simulink model "APF_CTL_VIS_Obs_2023a"  (R2023a)
settings: Solver=ode4  StartTime=0.0  StopTime=tsim  FixedStep=baseRate  RelTol=1e-6  AbsTol=1e-6
values from neighbouring files (symbols this model uses):
  A = [0 0 0 1 0 0 ... (first row only)    [CTL_NEW.m]    (also in UKF_SPOT.m = [1 0 0 dt 0 0)
  a = 25.028    [CTL_NEW.m]
  a1 = shape(1)    [Cardioid.m]    (also in Run_Initializer.m = 0.3)
  a2 = shape(2)    [Cardioid.m]    (also in Run_Initializer.m = 0.3)
  a3 = shape(3)    [Cardioid.m]    (also in Run_Initializer.m = 0.4)
  adadelta_epsilon = 1e-5    (= 1e-05)    [Run_Initializer.m]
  adadelta_gamma = 0.37    [Run_Initializer.m]
  adagrad_epsilon = 1e-8    (= 1e-08)    [Run_Initializer.m]
  adagrad_eta = 0.18    [Run_Initializer.m]
  adam_beta_1 = 0.99    [Run_Initializer.m]
  adam_beta_2 = 0.999    [Run_Initializer.m]
  adam_epsilon = 1e-2    (= 0.01)    [Run_Initializer.m]
  adam_eta = 0.0163    [Run_Initializer.m]
  adamax_beta_1 = 0.5    [Run_Initializer.m]
  adamax_beta_2 = 0.999    [Run_Initializer.m]
  adamax_eta = 0.014    [Run_Initializer.m]
  alpha_Black = 0.9    [UKF_SPOT.m]
  alpha_Blue = 0.9    [UKF_SPOT.m]
  Att_Mode = 0    [Run_Initializer.m]
  b1 = shape(4)    [Cardioid.m]    (also in Run_Initializer.m = 0.175)
  b2 = shape(5)    [Cardioid.m]    (also in Run_Initializer.m = 0.175)
  beta_Black = 2    [UKF_SPOT.m]
  beta_Blue = 20    [UKF_SPOT.m]
  Binv = inv(B)    [Run_Initializer.m]
  BLACK_end = [2, 1.4, deg2rad(368)]    [Run_Initializer.m]
  BLACK_ini = [2, 1.4, deg2rad(188), 0, 0, deg2rad(1.5)]    [Run_Initializer.m]
  BLUE_end = [1.3, 1.25, deg2rad(90)]    [Run_Initializer.m]
  BLUE_ini = [1.3, 1.25, deg2rad(270), 0, 0, deg2rad(-1.5)]    [Run_Initializer.m]
  drop_states_BLACK = BLACK_ini(1:3)    [Run_Initializer.m]
  drop_states_BLUE = BLUE_ini(1:3)    [Run_Initializer.m]
  drop_states_RED = RED_ini(1:3)    [Run_Initializer.m]
  dt = 0.01    [UKF_SPOT.m]
  end_time_black = 300    [Run_Initializer.m]
  end_time_blue = 300    [Run_Initializer.m]
  F_max = 0.22    [CTL_NEW.m]
  Gamma1_el = 0.12    [Run_Initializer.m]
  Gamma1_sh = 0.005    [Run_Initializer.m]
  Gamma1_wr = 0.025    [Run_Initializer.m]
  Gamma2_el = 5    [Run_Initializer.m]
  Gamma2_sh = 5    [Run_Initializer.m]
  Gamma2_wr = 5    [Run_Initializer.m]
  Gamma3_el = 10    [Run_Initializer.m]
  Gamma3_sh = 40    [Run_Initializer.m]
  Gamma3_wr = 40    [Run_Initializer.m]
  Gamma4_el = 0.039    [Run_Initializer.m]
  Gamma4_sh = 0.015    [Run_Initializer.m]
  Gamma4_wr = 0.029    [Run_Initializer.m]
  Gamma5_el = 800    [Run_Initializer.m]
  Gamma5_sh = 800    [Run_Initializer.m]
  Gamma5_wr = 800    [Run_Initializer.m]
  Gamma6_el = 0.000001    (= 1e-06)    [Run_Initializer.m]
  Gamma6_sh = 0.005    [Run_Initializer.m]
  Gamma6_wr = 0.02    [Run_Initializer.m]
  H = [1 0 0 0 0 0 ... (first row only)    [UKF_SPOT.m]
  home_states_BLACK = BLACK_ini(1:3)    [Run_Initializer.m]
  home_states_BLUE = BLUE_ini(1:3)    [Run_Initializer.m]
  home_states_RED = RED_ini(1:3)    [Run_Initializer.m]
  Hz = 0.01    [CTL_NEW.m]
  init_states_BLACK = BLACK_ini(1:3)    [Run_Initializer.m]
  init_states_BLUE = BLUE_ini(1:3)    [Run_Initializer.m]
  init_states_RED = RED_ini(1:3)    [Run_Initializer.m]
  J = IRED    [CTL_NEW.m]    (also in UKF_SPOT.m = 0.20184)
  k = lqr(A,B1,Q,R)    [CTL_NEW.m]
  k_1_0 = k(1,1)    [CTL_NEW.m]
  k_1_t_0 = k(3,3)    [CTL_NEW.m]
  k_2_0 = k(1,4)    [CTL_NEW.m]
  k_2_t_0 = k(3,6)    [CTL_NEW.m]
  K_a = diag([2 2 3.5])    [Run_Initializer.m]
  ka = 1    [Run_Initializer.m]
  Kd_elarm = 0.8    [Run_Initializer.m]
  Kd_sharm = 1.0    (= 1)    [Run_Initializer.m]
  Kd_t = 9.5    [CTL_NEW.m]    (also in Run_Initializer.m)
  Kd_wrarm = 0.6    [Run_Initializer.m]
  Kd_x = 28    [CTL_NEW.m]    (also in Run_Initializer.m)
  Kd_y = Kd_x    (= 28)    [CTL_NEW.m]    (also in Run_Initializer.m)
  Kp_elarm = 1.2    [Run_Initializer.m]
  Kp_sharm = 1.5    [Run_Initializer.m]
  Kp_t = 1    [CTL_NEW.m]    (also in Run_Initializer.m)
  Kp_wrarm = 2    [Run_Initializer.m]
  Kp_x = 3.5    [CTL_NEW.m]    (also in Run_Initializer.m)
  Kp_y = Kp_x    (= 3.5)    [CTL_NEW.m]    (also in Run_Initializer.m)
  kr = 2    [Run_Initializer.m]
  lambda1 = 0.4    [CTL_NEW.m]
  lambda12 = 0.4    [CTL_NEW.m]
  lambda12_t = 0.05    [CTL_NEW.m]
  lambda1_t = 0.05    [CTL_NEW.m]
  lambda2 = 0.4    [CTL_NEW.m]
  lambda2_t = 0.05    [CTL_NEW.m]
  lamda_Black = (alpha_Black^2)*(N + kappa_Black) - N    (= 15.06)    [UKF_SPOT.m]
  lamda_Blue = (alpha_Blue^2)*(N + kappa_Blue) - N    (= 6.96)    [UKF_SPOT.m]
  m = mRED    [CTL_NEW.m]    (also in UKF_SPOT.m = 11.21)
  method = 1    [UKF_SPOT.m]
  Method = 8    [Run_Initializer.m]
  momentum_eta = 0.7    [Run_Initializer.m]
  momentum_gamma = 0.7    [Run_Initializer.m]
  nesterov_eta = 0.6    [Run_Initializer.m]
  nesterov_gamma = 0.3    [Run_Initializer.m]
  Nmat = diag([1 1 1])    [Run_Initializer.m]
  p = 0.4    [CTL_NEW.m]
  P_b = diag([45 45 0])    [Run_Initializer.m]
  P_IC_Black = 0.2*eye(6)    [UKF_SPOT.m]
  P_IC_Blue = 0.2*eye(6)    [UKF_SPOT.m]
  p_t = 0.05    [CTL_NEW.m]
  psi = 1    [Run_Initializer.m]
  PWMFreq = 5    [Run_Initializer.m]
  Q = [w 0 0 0 0 0 ... (first row only)    [CTL_NEW.m]
  Q_a = diag([5, 5, 0])    [Run_Initializer.m]
  Q_b = diag([0.0125, 0.0125, 0.05])    [Run_Initializer.m]
  Q_Black = [0.0000005 0 0 0 0 0 ... (first row only)    [UKF_SPOT.m]
  Q_Blue = [0.000075 0 0 0 0 0 ... (first row only)    [UKF_SPOT.m]
  R = [r 0 0 ... (first row only)    [CTL_NEW.m]
  R_Black = [variance 0 0 ... (first row only)    [UKF_SPOT.m]
  R_Blue = [variance 0 0 ... (first row only)    [UKF_SPOT.m]
  r_hold = 0.427    [Run_Initializer.m]
  r_off = 0.165    [Run_Initializer.m]
  RED_ini = [2.7, 0.4, deg2rad(135+360), 0, 0, 0]    [Run_Initializer.m]
  Red_Rate = 0.025    [CTL_NEW.m]
  RMSprop_epsilon = 1e-8    (= 1e-08)    [Run_Initializer.m]
  RMSprop_eta = 0.025    [Run_Initializer.m]
  RMSprop_gamma = 0.9    [Run_Initializer.m]
  ... (+11 more)
undefined symbols (not defined in the file or in its folder): alpha, alpha_m, alphap, alphat, Am, b, b0, b3, baseRate, beta, Bm, c, Cm, d, DiscIntNeverNeededParam, Dm, drop_states_ARM, epsilon, F_Black_X_nominal, F_Black_Y_nominal, F_Blue_X_nominal, F_Blue_Y_nominal, F_red_X_nominal, F_red_Y_nominal, F_thrusters_BLACK, F_thrusters_BLUE, F_thrusters_RED, IBLACK, IBLUE, IDIST, IEE, IPROX, IRED, K, k1, k1t, k2, k2t, K_t, Kd_tb, Kd_tblue, Kd_tr, Kd_xb, Kd_xblue, Kd_xr, Kd_yb, Kd_yblue, Kd_yr, Kp_tb, Kp_tblue, Kp_tr, Kp_xb, Kp_xblue, Kp_xr, Kp_yb, Kp_yblue, Kp_yr, lamda ... (+34)
libraries: nvidiaSharedBlocks x10, MainLibrary x4, dspsigops x4, simulink x2, etargetslib x1
(part 14 of 15)

== matlab function APF_CTL_VIS_Obs_2023a/Phase #3: Experiment/Change RED Behavior/Sub-Phase #4/CTL/If Action Subsystem/Sat/MATLAB Function4 ==
  data: q2 input; u input; saturation output; F_max parameter; b parameter; m parameter; e parameter
function saturation = fcn(q2,u,F_max, b, m, e)

if u >= e
    u = e;
elseif u <= -1*e
    u = -1*e;
else
    u = u;
end

u = b*q2*m + u;

if u >= F_max
    u = F_max;
elseif u <= -1*F_max
    u = -1*F_max;
else
    u = u;
end

saturation = u;

== matlab function APF_CTL_VIS_Obs_2023a/Phase #3: Experiment/Change RED Behavior/Sub-Phase #4/CTL/If Action Subsystem/Sat/MATLAB Function5 ==
  data: q2 input; u input; saturation output; e parameter; T_max parameter; d parameter; J parameter
function saturation = fcn(q2,u,e, T_max, d, J)

if u >= e
    u = e;
elseif u <= -1*e
    u = -1*e;
else
    u = u;
end

u = d*q2*J + u;

if u >= T_max
    u = T_max;
elseif u <= -1*T_max
    u = -1*T_max;
else
    u = u;
end

saturation = u;

== matlab function APF_CTL_VIS_Obs_2023a/Phase #3: Experiment/Change RED Behavior/Sub-Phase #4/BLUE/Ryan's Transform ==
  data: Measurments input; Blue_Measurments_table_ref output; Red_States input; delta parameter
function Blue_Measurments_table_ref = RelitivetoTable(Measurments,Red_States,delta)
if anynan(Measurments)
    Blue_Measurments_table_ref = [NaN;NaN;NaN];
else

 Measurments(1,1) = Measurments(1);
 Measurments(2,1) = Measurments(2);
 Measurments = [Measurments; Red_States(3)];

%% This code is very scuffed, so I added lots of notes, feel free to change this
%% Size check
if size(Red_States,1) == 6 || size(Red_States,2) == 6
    Red_States = Red_States(1:3);
elseif size(Red_States,1) == 3 || size(Red_States,2) == 3
    % Nothin
else
    disp('Error with demensions of Red_States')
    disp('Please use 3 or 6 states')
    disp(':(')
end

if size(Measurments,1) == 3 || size(Measurments,2) == 3
    % Nothin
else
    disp('Error with demensions of Measurments')
    disp('VIS only gives 3 states, please only use 3 states')
    disp(':(')
end
Red_States(3) = mod(Red_States(3) + pi, 2*pi) - pi;

%% Rotation matrix scuffed (accounts for the location change of the docking cone) + Camera Offset of 3 deg
     c3 = [sin(Red_States(3) + delta*pi/180),  cos(Red_States(3) + delta*pi/180), 0;
          cos(Red_States(3) + delta*pi/180), -sin(Red_States(3) + delta*pi/180), 0;
          0,                     0,                    1];

%% Measurments in table ref frame
    Blue_Measurments_table_ref = c3*Measurments;

%% Vector addition
    Blue_Measurments_table_ref(1) = Blue_Measurments_table_ref(1) + Red_States(1); 
    Blue_Measurments_table_ref(2) =  -1*Blue_Measurments_table_ref(2) + Red_States(2); % Negative Y value accounting for "Left Hand Rule"

%% Angle addition
    Blue_Measurments_table_ref(3) = Red_States(3); % Setting this just to give an estimate

%% Wrapping Angle from -pi to pi
% Dont ask me why, its consistant with the SPOT inport from phasespace
% Dont belive me, look at this, angular velocity is being unwrapped, therefor, angle must be wrapped
% APF_Path_Planning_2023a/PhaseSpace Camera Code/Use Hardware to Obtain States
    % Black_Measurments_table_ref(3) = mod(Black_Measurments_table_ref(3) + pi, 2*pi) - pi;
end
end

== matlab function APF_CTL_VIS_Obs_2023a/Phase #3: Experiment/Change RED Behavior/Sub-Phase #4/CTL/Subsystem1/SAT_Angle1/MATLAB Function2 ==
  data: q2 input; q1 input; saturation output; c parameter; d parameter; J parameter
function saturation = fcn(q2,q1,c, d, J)

u = c*J*q1 + c*J*q2/d;

saturation = u;

== matlab function APF_CTL_VIS_Obs_2023a/Phase #3: Experiment/Change RED Behavior/Sub-Phase #4/CTL/Subsystem1/SAT_Angle1/MATLAB Function5 ==
  data: q2 input; u input; saturation output; e parameter; T_max parameter; d parameter; J parameter
function saturation = fcn(q2,u,e, T_max, d, J)

if u >= e
    u = e;
elseif u <= -1*e
    u = -1*e;
else
    u = u;
end

u = d*q2*J + u;

if u >= T_max
    u = T_max;
elseif u <= -1*T_max
    u = -1*T_max;
else
    u = u;
end

saturation = u;

== matlab function APF_CTL_VIS_Obs_2023a/Phase #3: Experiment/Change RED Behavior/Sub-Phase #4/CTL/Subsystem1/Subsystem/SAC Ctl/SAC Fns ==
  data: um input; u output; xm input; ey input; Ke_l input; Kx_l input; Ku_l input; Ke output; Kx output; Ku output; Kedot_l output; Kxdot_l output; Kudot_l output
function [u, Ke, Kx, Ku, Kedot_l, Kxdot_l, Kudot_l] = sac(um, xm, ey, Ke_l, Kx_l, Ku_l)

%%% Gains
gamma_l = [451300 0 0; 0 0 0; 0 0 0] ;
gamma_p = 3.5*[122500 0 0; 0 534500 0; 0 0 258000] ;
sigma_sac = 0.93 ;

%%% Ke
Kpe = ey*ey'*gamma_p(1,1) ;
Kedot_l = ey*ey'*gamma_l(1,1) - sigma_sac*Ke_l ;
Ke = Kpe + Ke_l ;

%%% Kx
Kpx = ey*xm'*gamma_p(2,2) ;
Kxdot_l = ey*xm'*gamma_l(2,2) ;
Kx = Kpx + Kx_l ;

%%% Ku
Kpu = ey*um'*gamma_p(3,3) ;
Kudot_l = ey*um'*gamma_l(3,3) ;
Ku = Kpu + Ku_l ;

%%% input
u = Ke*ey + Kx*xm + Ku*um ;

== matlab function APF_CTL_VIS_Obs_2023a/Phase #3: Experiment/Change RED Behavior/Sub-Phase #4/CTL/If Action Subsystem/DAC Controller3/Fx Gain Derivatives ==
  data: e_xdot input; k2_dot output; e_x input; k1_dot output; lambda1 parameter; lambda2 parameter; lambda12 parameter; p parameter
function [k2_dot, k1_dot]= fcn(e_xdot, e_x, lambda1, lambda2, lambda12, p)

k1_dot = -lambda1*p*e_x^2-(lambda1+p*lambda12)*e_x*e_xdot-lambda12*e_xdot^2;
k2_dot = -lambda12*p*e_x^2-(lambda12+p*lambda2)*e_x*e_xdot-lambda2*e_xdot^2;

== matlab function APF_CTL_VIS_Obs_2023a/Phase #3: Experiment/Change RED Behavior/Sub-Phase #4/CTL/If Action Subsystem/DAC Controller3/Fy Gain Derivatives ==
  data: k2_dot output; e_ydot input; e_y input; k1_dot output; lambda1 parameter; lambda2 parameter; lambda12 parameter; p parameter
function [k2_dot, k1_dot]= fcn(e_ydot, e_y, lambda1, lambda2, lambda12, p)

k1_dot = -lambda1*p*e_y^2-(lambda1+p*lambda12)*e_y*e_ydot-lambda12*e_ydot^2;
k2_dot = -lambda12*p*e_y^2-(lambda12+p*lambda2)*e_y*e_ydot-lambda2*e_ydot^2;

== matlab function APF_CTL_VIS_Obs_2023a/Phase #3: Experiment/Change RED Behavior/Sub-Phase #4/CTL/Subsystem1/SAT_Angle1/Torque Gain Derivatives ==
  data: e_t input; e_tdot input; k1_dot output size=1; k2_dot output size=1; lambda1_t parameter; lambda2_t parameter; lambda12_t parameter; p_t parameter
function [k1_dot, k2_dot]= fcn(e_t, e_tdot, lambda1_t, lambda2_t, lambda12_t, p_t)
k1_dot = -lambda1_t*p_t*e_t^2-(lambda1_t+p_t*lambda12_t)*e_t*e_tdot-lambda12_t*e_tdot^2;
k2_dot = -lambda12_t*p_t*e_t^2-(lambda12_t+p_t*lambda2_t)*e_t*e_tdot-lambda2_t*e_tdot^2;

== matlab function APF_CTL_VIS_Obs_2023a/Phase #3: Experiment/Change RED Behavior/Sub-Phase #4/CTL/If Action Subsystem/DAC Controller3/Torque Gain Derivatives ==
  data: e_t input; e_tdot input; k1_dot output size=1; k2_dot output size=1; lambda1_t parameter; lambda2_t parameter; lambda12_t parameter; p_t parameter
function [k1_dot, k2_dot]= fcn(e_t, e_tdot, lambda1_t, lambda2_t, lambda12_t, p_t)
k1_dot = -lambda1_t*p_t*e_t^2-(lambda1_t+p_t*lambda12_t)*e_t*e_tdot-lambda12_t*e_tdot^2;
k2_dot = -lambda12_t*p_t*e_t^2-(lambda12_t+p_t*lambda2_t)*e_t*e_tdot-lambda2_t*e_tdot^2;

== matlab function APF_CTL_VIS_Obs_2023a/Phase #3: Experiment/Change RED Behavior/Sub-Phase #4/BLUE/Subsystem/MATLAB Function ==
  data: u1 input; y output; u2 input
function y = fcn(u1,u2)
if abs(u1(1) - u2(1)) < 1e-10
    y = [NaN;NaN];
else
    y = u1;
end
if u1 < 1e-10
    y = [NaN;NaN];
end

== matlab function APF_CTL_VIS_Obs_2023a/Phase #3: Experiment/Change RED Behavior/Sub-Phase #4/BLUE/UKF_New/MATLAB Function2 ==
  data: no_IC output; States output; P_K output; Reject_Sum output; Reject output; Measurments input; Force input; States_k1 input; P_K1 input; lamda_Blue parameter; J parameter; m parameter; dt parameter; Q_Blue parameter; alpha_Blue parameter; beta_Blue parameter; H parameter; R_Blue parameter; thresh_Blue parameter; method parameter; Reject_sumk1 input; Reject_k1 input; thresh_Factor_Blue parameter
function [no_IC,States,P_K,Reject_Sum,Reject] = UKF(Measurments,Force,States_k1,P_K1, lamda_Blue, J, m, dt, Q_Blue, alpha_Blue, beta_Blue, H, R_Blue,thresh_Blue, method,Reject_sumk1,Reject_k1, thresh_Factor_Blue)
%% Block diagram got messy so i put it all in one block
if isempty(Force)
    Force = [0;0;0];
end

%% Inital position
if all(States_k1 == 0) || anynan(States_k1)
    if anynan(Measurments)
        States = NaN(6,1);
        no_IC = 1;
        P_K = P_K1;
        Reject_Sum = 0;
        Reject = 0;
    else
        States = [Measurments;zeros(3,1)];
        no_IC = 0;
        P_K = P_K1;
        Reject_Sum = 0;
        Reject = 0;
    end
else
    no_IC = 0;

    X_Cal = fcn1(States_k1,P_K1,lamda_Blue,method);
    
    X_Cal_k1 = fcn2(Force,X_Cal,J,m,dt);
    
    [w_m,w_c,X_tilda_k,P_K1] = fcn3(X_Cal_k1,lamda_Blue, Q_Blue, alpha_Blue, beta_Blue);
    
    [Z_Bar,Z_Cal] = fcn4(X_Cal_k1, w_m,H);
    
    [P_xz_k,P_z_k] = fcn5(Z_Bar,Z_Cal,w_c,X_tilda_k,X_Cal,R_Blue);
    
    K_k = fcn6(P_xz_k,P_z_k);
    
    Z_k = fcn7(Measurments);

    [thresh_Dynamic,Reject_Sum] = Dyn_Thresh(thresh_Blue,Reject_k1,thresh_Factor_Blue,Reject_sumk1);
    
    Reject = fcn8(Z_k,Z_Bar,P_z_k,thresh_Dynamic);
    
    States = fcn9(Z_k,Reject,X_tilda_k,Z_Bar,K_k);
    
    P_K = fcn10(P_K1,P_z_k,K_k,Reject);
end
end

function X_Cal = fcn1(x_tilda_k,P_k,lamda,method)
%% Calculate size of sigma var
sz = 6;
N = 2*sz + 1;
X_Cal = zeros(sz,N);

%% Calculate initial sigma point
X_Cal(:,1) = x_tilda_k;

%% Calculate sigma distance
sigma = (6 + lamda)*P_k;
sigma = Cholesky_Decomposition(sigma,method);

%% Calculate Sigma Points
% Positive points
for i = 2:1:((N-1)/2) + 1
    fill = zeros(size(x_tilda_k));
    fill(i-1,1) = sigma(i-1,i-1);
    X_Cal(:,i) = x_tilda_k + fill;
end
% Negative Points
j = 1;
for i = N + 1 - ((N-1)/2):1:N
    fill = zeros(size(x_tilda_k));
    fill(j,1) = sigma(j,j);
    X_Cal(:,i) = x_tilda_k - fill;
    j = j + 1;
end
end

function L = Cholesky_Decomposition(mat,method)

%% Getting size of matrix
[row,col] = size(mat);

%% Make sure matrix can be decomposed
if ~isequal(size(mat), size(mat'))
    error('Input matrix must be symmetric');
end

if any(eig(mat) <= 0)
    % error('Input matrix must be positive definite'); %% Added Error
    % Handling
    mat = NearPositiveDefinite(mat,method);
end

%% Pre allocating Space
L = zeros(row,col);

% Perform Cholesky decomposition
    for i = 1:col
        % Compute the diagonal element
        L(i, i) = sqrt(mat(i, i) - sum(L(i, 1:i-1).^2));
        
        % Compute the elements below the diagonal
        for j = i+1:col
            L(j, i) = (mat(j, i) - sum(L(j, 1:i-1).*L(i, 1:i-1))) / L(i, i);
        end
    end
end

function A_P = NearPositiveDefinite(A,method)
%% Method 1 (Symmetric Polar Factor)
%% Method 2 (Eigenvalue Recomposition)
    % enforce symmetry
    if isreal(A)
        B = 0.5*(A + A');
    else
        B = 0.5*(A + A');
        B = real(B) + 1i*hermSign(B).*imag(B);
    end

    if method == 1
        [~,~,U] = svd(B);
        H = U*U';
        A = (B + H)/2;

    elseif method == 2
        % Eigenvalue recomposition with modification for complex matrices
        [V,D] = eig(B);
        if isreal(A)
            D = max(real(D), 0); % Ensure real part of eigenvalues is non-negative
        else
            % For complex matrices, ensure positive semidefinite
            D = max(D, 0); % Ensure eigenvalues are non-negative
            V = real(V); % Take the real part of eigenvectors
        end
        A = real(V)*real(D)*real(V)'; % Now this really real product really should be really real right?
    else
        error('Please select proper method for Near Positive Definite Iteration')
    end

    % enforce symmetry again
    A_P = 0.5*(A + A');

    % Iteration
    i = 1;
    j = 0;
    max_iterations = 1000; % Maximum iterations allowed before increment starts increasing exponentially
    large_j_threshold = 500; % Threshold value for j to start increasing increment exponentially

    while i ~= 0
        [~,i] = chol(A_P);
        j = j + 1;
        if i ~= 0 % if close, add a multiple of the identity scaled by the smallest eigenvalue
            eig_min = min(eig(A_P));
            if j <= large_j_threshold
                increment = (-real(eig_min)*j.^2 + eps(real(eig_min)))*eye(size(A));
            else
                % Increase increment exponentially
                increment = (abs(real(eig_min))*j.^2 + eps(real(eig_min)))*exp(0.1*(j - large_j_threshold))*eye(size(A));
            end
            A_P = A_P + increment;
        end
        if j > max_iterations % If j exceeds the maximum allowed iterations, break the loop
            break;
        end
    end
end

function X_Cal_k1  = fcn2( F, X_Cal_k, J, m, dt)
%% Pre-Define
X_Cal_k1 = zeros(size(X_Cal_k));
%% System Dynamics
A = [eye(3), eye(3)*dt;
    zeros(3), eye(3)];

B = [eye(2)*(dt^2)/(2*m), zeros(2,1);
     0,0, (dt^2)/(2*J);
     eye(2)*(dt)/(m), zeros(2,1);
     0,0, (dt)/(J)];

%% State propigation
f = size(X_Cal_k,2);
for i = 1:1:f
    X_Cal_k1(:,i) = A*X_Cal_k(:,i) + B*F; 
end
end

function [w_m,w_c,X_tilda_k,P_K] = fcn3(X_Cal_k1,lamda, Q, alpha, beta)
%% Sigma weights
sz = size(X_Cal_k1,2);
N = 6;

%% For non modifyed variation
% w_0 = kappa/(N + kappa);
% w_i = 1/(2*(N + kappa));
% w = w_i*ones(1,N);
% w(1,1) = w_0;

%% Additional step - Sigma Points Weights
w_m_0 = lamda/(N + lamda);
w_c_0 = (lamda/(N + lamda)) + beta + (1 - alpha^2);
w_i = 1/(2*(N + lamda));

w = w_i*ones(1,sz-1);
w_m = [w_m_0, w];
w_c = [w_c_0, w];

w_m = diag(w_m);
w_c = diag(w_c);

%% State Prediction
X_tilda_k = X_Cal_k1*w_m;
X_tilda_k = sum(X_tilda_k,2);


%% Covariance Prediction
P_K = (X_Cal_k1 - X_tilda_k)*w_c*(X_Cal_k1 - X_tilda_k)' + Q;

end

function [Z_Bar,Z_Cal] = fcn4(x_Cal_k1, w_m,H)
%% calc Z_Cal
N = size(x_Cal_k1,2);
Z_Cal = zeros(3,N);
for i = 1:1:N
    Z_Cal(:,i) = H*x_Cal_k1(:,i);
end

%% Calc Z_Bar
Z_Bar = Z_Cal*w_m;
Z_Bar = sum(Z_Bar,2);
end

function [P_xz_k,P_z_k] = fcn5(Z_Bar,Z_Cal,w_c,x_tilda_k1,X_Cal,R)
%% calc P_z
P_z_k = (Z_Cal - Z_Bar)*w_c*(Z_Cal - Z_Bar)' + R;

%% calc P_xz
P_xz_k = (X_Cal - x_tilda_k1)*w_c*(Z_Cal - Z_Bar)';
end

function K_k = fcn6(P_xz_k,P_z_k)
K_k = (P_xz_k)*P_z_k';
end

function Z_k = fcn7(z_k)
    %% Assuming that all states are given or no states are given
    if anynan(z_k)
        Z_k = 1000*ones(3,1);
    else
    Z_k = z_k;
    end
end

function  Reject = fcn8(Z_k,Z_Bar,P_z_k,thresh)
%% Calc Mahalanobis Distance
D_square = (transpose(Z_k - Z_Bar))*P_z_k*(Z_k - Z_Bar);
% mahalanobis_d = sqrt(D_square);

%% Determine if data should be rejected
if D_square < thresh
    Reject = 0;
else
    Reject = 1;
end
end

function [x] = fcn9(z,Reject,X_tilda_k,z_bar,K_k)
%% State estimate
    if Reject == 0
        x = X_tilda_k + K_k*(z - z_bar);
    else
        x = X_tilda_k;
    end
end

function P_K = fcn10(P_k1,P_z_k,K_k,Reject)
if Reject == 0
    P_K = P_k1 - (K_k*P_z_k)*K_k';
else
    P_K = P_k1;
end
end


function [thresh_Dynamic,Reject_Sum] = Dyn_Thresh(thresh_Black,Reject_k1,thresh_Factor_Black,Reject_sumk1)
if Reject_k1 == 1    
    Reject_Sum = Reject_sumk1 + 1;
    thresh_Dynamic = thresh_Black + Reject_Sum*thresh_Factor_Black;
else 
    Reject_Sum = 0;
    thresh_Dynamic = thresh_Black;
end
end

== matlab function APF_CTL_VIS_Obs_2023a/Thruster Control Code/Change RED Behavior/Calculate Thruster ON//OFF/MATLAB Function11 ==
  data: H output; thruster_dist2CG_RED parameter; F_red_X_nominal parameter; thrust_decay_factor input; F_red_Y_nominal parameter
function H   = MakeHWithDecay(thruster_dist2CG_RED,F_red_X_nominal, thrust_decay_factor, F_red_Y_nominal)


adjusted_thruster_dist2CG_RED = [thruster_dist2CG_RED(1);
                                 thruster_dist2CG_RED(2);
                                 thruster_dist2CG_RED(3);
                                 thruster_dist2CG_RED(4);
                                 thruster_dist2CG_RED(5);
                                 thruster_dist2CG_RED(6);
                                 thruster_dist2CG_RED(7);
                                 thruster_dist2CG_RED(8)];
                                 


Vec1 = [ -1
         -1
          0 
          0
          1
          1
          0
          0 ];
      
Vec2 = [  0
          0
          1
          1
          0
          0
         -1
         -1 ];
     
Vec3 = adjusted_thruster_dist2CG_RED./1000;

Mat1 = [Vec1, Vec2, Vec3]';

F_thrusters_RED = [F_red_X_nominal*thrust_decay_factor; F_red_X_nominal*thrust_decay_factor; F_red_Y_nominal*thrust_decay_factor; F_red_Y_nominal*thrust_decay_factor; F_red_X_nominal*thrust_decay_factor; F_red_X_nominal*thrust_decay_factor; F_red_Y_nominal*thrust_decay_factor; F_red_Y_nominal*thrust_decay_factor];

Mat2 = diag((F_thrusters_RED./2));

H    = Mat1*Mat2;

end

== matlab function APF_CTL_VIS_Obs_2023a/Phase #3: Experiment/Change RED Behavior/Sub-Phase #4/BLACK/Subsystem/MATLAB Function ==
  data: u1 input; y output; u2 input
function y = fcn(u1,u2)
if abs(u1(1) - u2(1)) < 1e-10
    y = [NaN;NaN;NaN];
else
    y = u1;
end

== matlab function APF_CTL_VIS_Obs_2023a/Simulate Plant Dynamics/RED and ARM Dynamics/RED + ARM/RED + ARM Dynamics/Inertia Function 1 ==
  data: mRED parameter; IRED parameter; Phi parameter; b0 parameter; a1 parameter; b1 parameter; a2 parameter; b2 parameter; a3 parameter; b3 parameter; mPROX parameter; mDIST parameter; mEE parameter; IPROX parameter; IDIST parameter; InertiaS output; x input; IEE parameter
function InertiaS = InertiaFunc3LINK(mRED, IRED, Phi, b0, a1, b1, a2, b2, a3, b3, mPROX, mDIST, mEE, IPROX, IDIST, x, IEE)

    q0 = x(3);
    q1 = x(4);
    q2 = x(5);
    q3 = x(6);
    
    t2 = a1+b1;
    t3 = a1.*mPROX;
    t4 = mDIST.*t2;
    t5 = mEE.*t2;
    t6 = q0+q1;
    t7 = cos(t6);
    t8 = t3+t4+t5;
    t9 = a2.*mDIST;
    t10 = a2+b2;
    t11 = mEE.*t10;
    t12 = q0+q1+q2;
    t13 = cos(t12);
    t14 = t9+t11;
    t15 = q0+q1+q2+q3;
    t16 = cos(t15);
    t17 = mRED+mPROX+mDIST+mEE;
    t18 = b0.*mPROX;
    t19 = b0.*mDIST;
    t20 = b0.*mEE;
    t21 = t18+t19+t20;
    t22 = (pi/2-Phi)+q0;
    t23 = sin(t6);
    t24 = sin(t12);
    t25 = sin(t15);
    t26 = a2.*mEE;
    t27 = b2.*mEE;
    t28 = t9+t26+t27;
    t29 = sin(t22);
    t86 = t7.*t8;
    t87 = t13.*t14;
    t88 = a3.*mEE.*t16;
    t30 = -t86-t87-t88-t21.*t29;
    t31 = cos(t22);
    t32 = t21.*t31;
    t89 = t8.*t23;
    t90 = t14.*t24;
    t91 = a3.*mEE.*t25;
    t33 = t32-t89-t90-t91;
    t34 = a1.^2;
    t35 = a2.^2;
    t36 = b0.^2;
    t37 = b1.^2;
    t38 = a1.*a2.*mDIST.*2.0;
    t39 = a1.*a2.*mEE.*2.0;
    t40 = a2.*b1.*mDIST.*2.0;
    t41 = a1.*b2.*mEE.*2.0;
    t42 = a2.*b1.*mEE.*2.0;
    t43 = b1.*b2.*mEE.*2.0;
    t44 = t38+t39+t40+t41+t42+t43;
    t45 = cos(q2);
    t46 = t44.*t45;
    t47 = a2.*a3.*mEE.*2.0;
    t48 = a3.*b2.*mEE.*2.0;
    t49 = t47+t48;
    t50 = cos(q3);
    t51 = t49.*t50;
    t52 = a1.*a3.*mEE.*2.0;
    t53 = a3.*b1.*mEE.*2.0;
    t54 = t52+t53;
    t55 = q2+q3;
    t56 = cos(t55);
    t57 = t54.*t56;
    t58 = (pi/2-Phi)-q1;
    t59 = sin(t58);
    t60 = -(pi/2-Phi)+q1+q2;
    t61 = sin(t60);
    t62 = -(pi/2-Phi)+q1+q2+q3;
    t63 = sin(t62);
    t64 = mPROX.*t34;
    t65 = mDIST.*t34;
    t66 = mEE.*t34;
    t67 = mDIST.*t35;
    t68 = mEE.*t35;
    t69 = a3.^2;
    t70 = mEE.*t69;
    t71 = mDIST.*t37;
    t72 = mEE.*t37;
    t73 = b2.^2;
    t74 = mEE.*t73;
    t75 = a1.*b1.*mDIST.*2.0;
    t76 = a1.*b1.*mEE.*2.0;
    t77 = a2.*b2.*mEE.*2.0;
    t78 = a2.*b0.*mDIST;
    t79 = a2.*b0.*mEE;
    t80 = b0.*b2.*mEE;
    t81 = t78+t79+t80;
    t82 = a1.*a3.*mEE;
    t83 = a3.*b1.*mEE;
    t84 = t82+t83;
    t85 = t56.*t84;
    t92 = a1.*b0.*mPROX;
    t93 = a1.*b0.*mDIST;
    t94 = a1.*b0.*mEE;
    t95 = b0.*b1.*mDIST;
    t96 = b0.*b1.*mEE;
    t97 = t92+t93+t94+t95+t96;
    t98 = t59.*t97;
    t112 = t61.*t81;
    t113 = a3.*b0.*mEE.*t63;
    t99 = IPROX+IDIST+IEE+t46+t51+t57+t64+t65+t66+t67+t68+t70+t71+t72+t74+t75+t76+t77+t98-t112-t113;
    t100 = a1.*a2.*mDIST;
    t101 = a1.*a2.*mEE;
    t102 = a2.*b1.*mDIST;
    t103 = a1.*b2.*mEE;
    t104 = a2.*b1.*mEE;
    t105 = b1.*b2.*mEE;
    t106 = t100+t101+t102+t103+t104+t105;
    t107 = t45.*t106;
    t108 = a2.*a3.*mEE;
    t109 = a3.*b2.*mEE;
    t110 = t108+t109;
    t111 = t50.*t110;
    t114 = IDIST+IEE+t51+t67+t68+t70+t74+t77+t85+t107;
    t115 = IEE+t70+t85+t111;
    t116 = IEE+t70+t111;
    InertiaS = reshape([t17,0.0,t30,-t86-t87-t88,-t88-t13.*t28,-t88,0.0,t17,t33,-t89-t90-t91,-t91-t24.*t28,-t91,t30,t33,IRED+IPROX+IDIST+IEE+t46+t51+t57+t64+t65+t66+t67+t68+t70+t71+t72+t74+t75+t76+t77+t59.*(a1.*b0.*mPROX.*2.0+a1.*b0.*mDIST.*2.0+a1.*b0.*mEE.*2.0+b0.*b1.*mDIST.*2.0+b0.*b1.*mEE.*2.0)+mPROX.*t36+mDIST.*t36+mEE.*t36-t61.*(a2.*b0.*mDIST.*2.0+a2.*b0.*mEE.*2.0+b0.*b2.*mEE.*2.0)-a3.*b0.*mEE.*t63.*2.0,t99,IDIST+IEE+t51+t67+t68+t70+t74+t77+t85+t107-t112-t113,IEE+t70+t85+t111-t113,-t7.*t8-t13.*t14-a3.*mEE.*t16,-t8.*t23-t14.*t24-a3.*mEE.*t25,t99,IPROX+IDIST+IEE+t46+t51+t57+t64+t65+t66+t67+t68+t70+t71+t72+t74+t75+t76+t77,t114,t115,-t13.*t28-a3.*mEE.*t16,-t24.*t28-a3.*mEE.*t25,IDIST+IEE+t51+t67+t68+t70+t74+t77+t85+t107-t61.*t81-a3.*b0.*mEE.*t63,t114,IDIST+IEE+t51+t67+t68+t70+t74+t77,t116,-a3.*mEE.*t16,-a3.*mEE.*t25,IEE+t70+t85+t111-a3.*b0.*mEE.*t63,t115,t116,IEE+t70],[6,6]);
end

== matlab function APF_CTL_VIS_Obs_2023a/Thruster Control Code/Change RED Behavior/Calculate Thruster ON//OFF/MATLAB Function7 ==
  data: H output; thruster_dist2CG_RED parameter; F_red_X_nominal parameter; thrust_decay_factor input; F_red_Y_nominal parameter
function H   = MakeHWithDecay(thruster_dist2CG_RED,F_red_X_nominal, thrust_decay_factor, F_red_Y_nominal)


adjusted_thruster_dist2CG_RED = [thruster_dist2CG_RED(1);
                                 thruster_dist2CG_RED(2);
                                 thruster_dist2CG_RED(3);
                                 thruster_dist2CG_RED(4);
                                 thruster_dist2CG_RED(5);
                                 thruster_dist2CG_RED(6);
                                 thruster_dist2CG_RED(7);
                                 thruster_dist2CG_RED(8)];
                                 


Vec1 = [ -1
         -1
          0 
          0
          1
          1
          0
          0 ];
      
Vec2 = [  0
          0
          1
          1
          0
          0
         -1
         -1 ];
     
Vec3 = adjusted_thruster_dist2CG_RED./1000;

Mat1 = [Vec1, Vec2, Vec3]';

F_thrusters_RED = [F_red_X_nominal*thrust_decay_factor; F_red_X_nominal*thrust_decay_factor; F_red_Y_nominal*thrust_decay_factor; F_red_Y_nominal*thrust_decay_factor; F_red_X_nominal*thrust_decay_factor; F_red_X_nominal*thrust_decay_factor; F_red_Y_nominal*thrust_decay_factor; F_red_Y_nominal*thrust_decay_factor];

Mat2 = diag((F_thrusters_RED));

H    = Mat1*Mat2;

end

== matlab function APF_CTL_VIS_Obs_2023a/Simulate Plant Dynamics/BLACK Dynamics/BLACK Dynamics Model/MATLAB Function ==
  data: control_inputs input; x_ddot output; mBLACK parameter; IBLACK parameter
function x_ddot = BLACK_dynamics(control_inputs, mBLACK, IBLACK)

%#codegen
% Fully define the size of x_ddot() for code generation:
x_ddot     = zeros(3,1);

% Extract the control inputs from the control_input vector:
Fx        = control_inputs(1);              % [N]
Fy        = control_inputs(2);              % [N]
Tz        = control_inputs(3);              % [N.m]

% Calculate the state acceleration vector:
x_ddot(1) = Fx/mBLACK;                      % [m/s^2]
x_ddot(2) = Fy/mBLACK;                      % [m/s^2]
x_ddot(3) = Tz/IBLACK;                      % [rad/s^2]

end

== matlab function APF_CTL_VIS_Obs_2023a/Simulate Plant Dynamics/BLUE Dynamics/BLUE  Dynamics Model/MATLAB Function ==
  data: control_inputs input; x_ddot output; mBLUE parameter; IBLUE parameter
function x_ddot = BLUE_dynamics(control_inputs, mBLUE, IBLUE)%#codegen
% Fully define the size of x_ddot() for code generation:
x_ddot     = zeros(3,1);

% Extract the control inputs from the control_input vector:
Fx        = control_inputs(1);              % [N]
Fy        = control_inputs(2);              % [N]
Tz        = control_inputs(3);              % [N.m]

% Calculate the state acceleration vector:
x_ddot(1) = Fx/mBLUE;                      % [m/s^2]
x_ddot(2) = Fy/mBLUE;                      % [m/s^2]
x_ddot(3) = Tz/IBLUE;                      % [rad/s^2]

end

== matlab function APF_CTL_VIS_Obs_2023a/Simulate Plant Dynamics/BLUE Dynamics/Sample and Hold Data to Match PhaseSpace (BLUE)/MATLAB Function ==
  data: TIME input; y output; SERVER input
function y = fcn(TIME, SERVER)

if mod(TIME,SERVER) == 0
    y = 1;
else
    y = 0;
end

== matlab function APF_CTL_VIS_Obs_2023a/Simulate Plant Dynamics/RED and ARM Dynamics/RED Only/RED Dynamics/RED Dynamics Model/MATLAB Function ==
  data: control_inputs input; x_ddot output; mRED parameter; IRED parameter
    function x_ddot = RED_dynamics(control_inputs, mRED, IRED)
    
        %#codegen
        % Fully define the size of x_ddot() for code generation:
        x_ddot     = zeros(3,1);
        
        % Extract the servicer model parameters from the model_param vector defined
        % in initialize.m:
        
        % Extract the control inputs from the control_input vector:
        Fx        = control_inputs(1);              % [N]
        Fy        = control_inputs(2);              % [N]
        Tz        = control_inputs(3);              % [N.m]
        
        % Calculate the state acceleration vector:
        x_ddot(1) = Fx/mRED;                      % [m/s^2]
        x_ddot(2) = Fy/mRED;                      % [m/s^2]
        x_ddot(3) = Tz/IRED;                      % [rad/s^2]
    
    end

== matlab function APF_CTL_VIS_Obs_2023a/Phase #2: Initial Position/Change RED Behavior/MATLAB Function2 ==
  data: error input; error_d input; u output; K_lqr parameter
function u = fcn(error,error_d,K_lqr)




u = K_lqr*([error(1);error(2);error(3);error_d(1);error_d(2);error_d(3)]);

end

== matlab function APF_CTL_VIS_Obs_2023a/Phase #3: Experiment/Change RED Behavior/Sub-Phase #4/GDC/APF/GDC/MATLAB Function ==
  data: phi_tot output; phi_tot_grad output; state_red input; state_black input size=[6 1]; state_blue input; u output size=[3 1]; shape parameter; ka parameter; kr parameter; Q_a parameter; Q_b parameter; P_b parameter; r_hold parameter; Binv parameter; K_a parameter; psi parameter; sigma parameter; r_off parameter; Nmat parameter; state_desired output; IsBlue input
function [phi_tot,phi_tot_grad,u,state_desired] = fcn(state_red,state_black,state_blue,shape,ka,kr,Q_a,Q_b,P_b,r_hold,Binv,K_a,psi,sigma,r_off,Nmat,IsBlue)

[phi_tot,phi_tot_grad,u,state_desired] = APF_func_Maybe_Obstacle(state_red,state_black,state_blue,shape,ka,kr,Q_a,Q_b,P_b,r_hold,Binv,K_a,psi,sigma,r_off,Nmat,IsBlue);

== matlab function APF_CTL_VIS_Obs_2023a/Thruster Control Code/Change BLACK Behavior/Calculate Thruster ON//OFF/MATLAB Function ==
  data: H output; thruster_dist2CG_BLACK parameter; F_thrusters_BLACK parameter
function H = MakeH(thruster_dist2CG_BLACK,F_thrusters_BLACK)

Vec1 = [ -1
         -1
          0 
          0
          1
          1
          0
          0 ];
      
Vec2 = [  0
          0
          1
          1
          0
          0
         -1
         -1 ];
     
Vec3 = thruster_dist2CG_BLACK./1000;

Mat1 = [Vec1, Vec2, Vec3]';

Mat2 = diag((F_thrusters_BLACK./2));

H    = Mat1*Mat2;

end

== matlab function APF_CTL_VIS_Obs_2023a/Thruster Control Code/Change BLUE Behavior/Calculate Thruster ON//OFF/MATLAB Function1 ==
  data: H output; thruster_dist2CG_BLUE parameter; F_Blue_X_nominal parameter; thrust_decay_factor input; F_Blue_Y_nominal parameter
function H   = MakeHWithDecay(thruster_dist2CG_BLUE,F_Blue_X_nominal, thrust_decay_factor, F_Blue_Y_nominal)


adjusted_thruster_dist2CG_BLUE = [thruster_dist2CG_BLUE(1);
                                 thruster_dist2CG_BLUE(2);
                                 thruster_dist2CG_BLUE(3);
                                 thruster_dist2CG_BLUE(4);
                                 thruster_dist2CG_BLUE(5);
                                 thruster_dist2CG_BLUE(6);
                                 thruster_dist2CG_BLUE(7);
                                 thruster_dist2CG_BLUE(8)];
                                 


Vec1 = [ -1
         -1
          0 
          0
          1
          1
          0
          0 ];
      
Vec2 = [  0
          0
          1
          1
          0
          0
         -1
         -1 ];
     
Vec3 = adjusted_thruster_dist2CG_BLUE./1000;

Mat1 = [Vec1, Vec2, Vec3]';

F_thrusters_BLUE = [F_Blue_X_nominal*thrust_decay_factor; F_Blue_X_nominal*thrust_decay_factor; F_Blue_Y_nominal*thrust_decay_factor; F_Blue_Y_nominal*thrust_decay_factor; F_Blue_X_nominal*thrust_decay_factor; F_Blue_X_nominal*thrust_decay_factor; F_Blue_Y_nominal*thrust_decay_factor; F_Blue_Y_nominal*thrust_decay_factor];

Mat2 = diag((F_thrusters_BLUE));

H    = Mat1*Mat2;

end

== matlab function APF_CTL_VIS_Obs_2023a/Thruster Control Code/Change BLUE Behavior/Calculate Thruster ON//OFF/MATLAB Function2 ==
  data: ThrustPer_Final output; ThrustPer input; PWMFreq parameter
function ThrustPer_Final  = ThrusterSat(ThrustPer, PWMFreq)

    ValveTime       = 0.007;
    TControl        = 1/PWMFreq;

    ThrustPer_Final = zeros(8,1);
    
    if max(ThrustPer) > 1
        ThrustPer_Sat = ThrustPer/max(ThrustPer);
    else
        ThrustPer_Sat = ThrustPer;
    end
    
    for i = 1:8
        if ThrustPer_Sat(i) > ValveTime/TControl 
            ThrustPer_Final(i) = ThrustPer_Sat(i);
        else
            ThrustPer_Final(i) = 0;
        end
    end


end

== matlab function APF_CTL_VIS_Obs_2023a/Thruster Control Code/Change BLACK Behavior/Calculate Thruster ON//OFF/Rotate Forces to Inertial/Create Rotation Matrix ==
  data: Rz input; C_Ib output
function C_Ib = RotateFrame(Rz)

C_bI = [  cos(Rz) sin(Rz)
         -sin(Rz) cos(Rz) ];

C_Ib = inv(C_bI);

end

== matlab function APF_CTL_VIS_Obs_2023a/Thruster Control Code/Change BLACK Behavior/Rotate Forces to Body/Create Rotation Matrix ==
  data: Rz input; C_bI output
function C_bI = RotateFrame(Rz)

C_bI = [  cos(Rz) sin(Rz)
         -sin(Rz) cos(Rz) ];

end

== matlab function APF_CTL_VIS_Obs_2023a/Thruster Control Code/Change BLUE Behavior/Calculate Thruster ON//OFF/MATLAB Function ==
  data: H output; thruster_dist2CG_BLUE parameter; F_thrusters_BLUE parameter
function H = MakeH(thruster_dist2CG_BLUE,F_thrusters_BLUE)

Vec1 = [ -1
         -1
          0 
          0
          1
          1
          0
          0 ];
      
Vec2 = [  0
          0
          1
          1
          0
          0
         -1
         -1 ];
     
Vec3 = thruster_dist2CG_BLUE./1000;

Mat1 = [Vec1, Vec2, Vec3]';

Mat2 = diag((F_thrusters_BLUE./2));

H    = Mat1*Mat2;

end

== matlab function APF_CTL_VIS_Obs_2023a/Thruster Control Code/Change BLACK Behavior/Calculate Thruster ON//OFF/MATLAB Function1 ==
  data: ThrustPer_Final output; ThrustPer input; PWMFreq parameter
function ThrustPer_Final  = ThrusterSat(ThrustPer, PWMFreq)

    ValveTime       = 0.007;
    TControl        = 1/PWMFreq;

    ThrustPer_Final = zeros(8,1);
    
    if max(ThrustPer) > 1
        ThrustPer_Sat = ThrustPer/max(ThrustPer);
    else
        ThrustPer_Sat = ThrustPer;
    end
    
    for i = 1:8
        if ThrustPer_Sat(i) > ValveTime/TControl 
            ThrustPer_Final(i) = ThrustPer_Sat(i);
        else
            ThrustPer_Final(i) = 0;
        end
    end


end

== matlab function APF_CTL_VIS_Obs_2023a/Phase #3: Experiment/Change RED Behavior/Sub-Phase #4/GDC/APF/GDC/Subsystem1/Momentum/Momentum ==
  data: state_red input; phi_tot_grad input; v_prev input; path output size=3; v output size=3; momentum_eta parameter; momentum_gamma parameter
function [path, v] = momentum(state_red, phi_tot_grad, v_prev, momentum_eta, momentum_gamma)

% gamma = 0.9
v = -momentum_gamma.*v_prev-momentum_eta.*phi_tot_grad;
path = [state_red(1); state_red(2); state_red(3)] + v;

== matlab function APF_CTL_VIS_Obs_2023a/Thruster Control Code/Change BLUE Behavior/Calculate Thruster ON//OFF/Rotate Forces to Inertial/Create Rotation Matrix ==
  data: Rz input; C_Ib output
function C_Ib = RotateFrame(Rz)

C_bI = [  cos(Rz) sin(Rz)
         -sin(Rz) cos(Rz) ];

C_Ib = inv(C_bI);

end

== matlab function APF_CTL_VIS_Obs_2023a/Thruster Control Code/Change BLUE Behavior/Rotate Forces to Body/Create Rotation Matrix ==
  data: Rz input; C_bI output
function C_bI = RotateFrame(Rz)

C_bI = [  cos(Rz) sin(Rz)
         -sin(Rz) cos(Rz) ];

end

== matlab function APF_CTL_VIS_Obs_2023a/Phase #2: Initial Position/Change BLACK Behavior/Hough Control/MATLAB Function2 ==
  data: Oy output; z input; Ox output
function [Oy, Ox]   = C3( z )
%C3 gives the rotation matrix about the z-axis for an angle 'z'
%   z - the angle about the z-axis which you rotate
%   A - the rotation matrix

Ox = [cos(z) sin(z); -sin(z) cos(z)]*[1;0];
Oy = [cos(z) sin(z); -sin(z) cos(z)]*[0;1];
end

== matlab function APF_CTL_VIS_Obs_2023a/Phase #2: Initial Position/Change BLACK Behavior/Hough Control/MATLAB Function3 ==
  data: z input; Ox output
function Ox    = C3( z )
%C3 gives the rotation matrix about the z-axis for an angle 'z'
%   z - the angle about the z-axis which you rotate
%   A - the rotation matrix

Ox = [cos(z) sin(z); -sin(z) cos(z)]*[1;0];
end

== matlab function APF_CTL_VIS_Obs_2023a/Phase #2: Initial Position/Change BLACK Behavior/Hough Control/MATLAB Function4 ==
  data: Oy input; e_out output; e_in input
function e_out = fcn(Oy, e_in)

a = sign(Oy'*e_in);
e_out = -a*norm(e_in);

== matlab function APF_CTL_VIS_Obs_2023a/Phase #2: Initial Position/Change BLUE Behavior/Hough Control/MATLAB Function2 ==
  data: Oy output; z input; Ox output
function [Oy, Ox]   = C3( z )
%C3 gives the rotation matrix about the z-axis for an angle 'z'
%   z - the angle about the z-axis which you rotate
%   A - the rotation matrix

Ox = [cos(z) sin(z); -sin(z) cos(z)]*[1;0];
Oy = [cos(z) sin(z); -sin(z) cos(z)]*[0;1];
end

== matlab function APF_CTL_VIS_Obs_2023a/Thruster Control Code/Change RED Behavior/Rotate Forces to Body/Create Rotation Matrix ==
  data: Rz input; C_bI output
function C_bI = RotateFrame(Rz)

C_bI = [  cos(Rz) sin(Rz)
         -sin(Rz) cos(Rz) ];

end

== matlab function APF_CTL_VIS_Obs_2023a/Phase #2: Initial Position/Change BLUE Behavior/Hough Control/MATLAB Function3 ==
  data: z input; Ox output
function Ox    = C3( z )
%C3 gives the rotation matrix about the z-axis for an angle 'z'
%   z - the angle about the z-axis which you rotate
%   A - the rotation matrix

Ox = [cos(z) sin(z); -sin(z) cos(z)]*[1;0];
end

== matlab function APF_CTL_VIS_Obs_2023a/Phase #2: Initial Position/Change BLUE Behavior/Hough Control/MATLAB Function4 ==
  data: Oy input; e_out output; e_in input
function e_out = fcn(Oy, e_in)

a = sign(Oy'*e_in);
e_out = -a*norm(e_in);

== matlab function APF_CTL_VIS_Obs_2023a/Phase #2: Initial Position/Change RED Behavior/Hough Control/MATLAB Function2 ==
  data: Oy output; z input; Ox output
function [Oy, Ox]   = C3( z )
%C3 gives the rotation matrix about the z-axis for an angle 'z'
%   z - the angle about the z-axis which you rotate
%   A - the rotation matrix

Ox = [cos(z) sin(z); -sin(z) cos(z)]*[1;0];
Oy = [cos(z) sin(z); -sin(z) cos(z)]*[0;1];
end

== matlab function APF_CTL_VIS_Obs_2023a/Phase #2: Initial Position/Change RED Behavior/Hough Control/MATLAB Function3 ==
  data: z input; Ox output
function Ox    = C3( z )
%C3 gives the rotation matrix about the z-axis for an angle 'z'
%   z - the angle about the z-axis which you rotate
%   A - the rotation matrix

Ox = [cos(z) sin(z); -sin(z) cos(z)]*[1;0];
end

== matlab function APF_CTL_VIS_Obs_2023a/Phase #2: Initial Position/Change RED Behavior/Hough Control/MATLAB Function4 ==
  data: Oy input; e_out output; e_in input
function e_out = fcn(Oy, e_in)

a = sign(Oy'*e_in);
e_out = -a*norm(e_in);

== matlab function APF_CTL_VIS_Obs_2023a/Phase #3: Experiment/Change BLACK Behavior/Sub-Phase #4/BLACK_RzD/Wrap1/MATLAB Function ==
  data: u input; wrappedAngle output
function wrappedAngle = wrapAngle(u)

wrappedAngle = atan2(sin(u),cos(u));

end

== matlab function APF_CTL_VIS_Obs_2023a/Phase #3: Experiment/Change RED Behavior/Sub-Phase #4/GDC/Switch logic/Switch logic ==
  data: NO_IC input; Phase output; k1 input; Time_Look parameter; k output; Hz parameter
function [Phase,k] = fcn(NO_IC,k1,Time_Look,Hz)
%% Time Look is in seconds
if NO_IC == 1 
    Phase = 1;
    k = 0;
else
    k = k1 + 1;
    if k <= Time_Look/Hz
        Phase = 2;
    else
        Phase = 3;
    end
end
end

== matlab function APF_CTL_VIS_Obs_2023a/Phase #3: Experiment/Change BLACK Behavior/Sub-Phase #4/Hough Control/MATLAB Function2 ==
  data: Oy output; z input; Ox output
function [Oy, Ox]   = C3( z )
%C3 gives the rotation matrix about the z-axis for an angle 'z'
%   z - the angle about the z-axis which you rotate
%   A - the rotation matrix

Ox = [cos(z) sin(z); -sin(z) cos(z)]*[1;0];
Oy = [cos(z) sin(z); -sin(z) cos(z)]*[0;1];
end

== matlab function APF_CTL_VIS_Obs_2023a/Phase #3: Experiment/Change RED Behavior/Sub-Phase #2 /RED_Rz Desired/Wrap/MATLAB Function ==
  data: u input; wrappedAngle output
function wrappedAngle = wrapAngle(u)

wrappedAngle = atan2(sin(u),cos(u));

end

== matlab function APF_CTL_VIS_Obs_2023a/Phase #3: Experiment/Change BLACK Behavior/Sub-Phase #4/Hough Control/MATLAB Function3 ==
  data: z input; Ox output
function Ox    = C3( z )
%C3 gives the rotation matrix about the z-axis for an angle 'z'
%   z - the angle about the z-axis which you rotate
%   A - the rotation matrix

Ox = [cos(z) sin(z); -sin(z) cos(z)]*[1;0];
end

== matlab function APF_CTL_VIS_Obs_2023a/Phase #3: Experiment/Change BLACK Behavior/Sub-Phase #1/BLACK_Rz Desired/Wrap1/MATLAB Function ==
  data: u input; wrappedAngle output
function wrappedAngle = wrapAngle(u)

wrappedAngle = atan2(sin(u),cos(u));

end

== matlab function APF_CTL_VIS_Obs_2023a/Phase #3: Experiment/Change BLACK Behavior/Sub-Phase #1/Hough Control/MATLAB Function2 ==
  data: Oy output; z input; Ox output
function [Oy, Ox]   = C3( z )
%C3 gives the rotation matrix about the z-axis for an angle 'z'
%   z - the angle about the z-axis which you rotate
%   A - the rotation matrix

Ox = [cos(z) sin(z); -sin(z) cos(z)]*[1;0];
Oy = [cos(z) sin(z); -sin(z) cos(z)]*[0;1];
end

== matlab function APF_CTL_VIS_Obs_2023a/Phase #3: Experiment/Change BLACK Behavior/Sub-Phase #1/Hough Control/MATLAB Function3 ==
  data: z input; Ox output
function Ox    = C3( z )
%C3 gives the rotation matrix about the z-axis for an angle 'z'
%   z - the angle about the z-axis which you rotate
%   A - the rotation matrix

Ox = [cos(z) sin(z); -sin(z) cos(z)]*[1;0];
end

== matlab function APF_CTL_VIS_Obs_2023a/Phase #3: Experiment/Change BLUE Behavior/Sub-Phase #1/Hough Control/MATLAB Function2 ==
  data: Oy output; z input; Ox output
function [Oy, Ox]   = C3( z )
%C3 gives the rotation matrix about the z-axis for an angle 'z'
%   z - the angle about the z-axis which you rotate
%   A - the rotation matrix

Ox = [cos(z) sin(z); -sin(z) cos(z)]*[1;0];
Oy = [cos(z) sin(z); -sin(z) cos(z)]*[0;1];
end

== matlab function APF_CTL_VIS_Obs_2023a/Phase #3: Experiment/Change BLUE Behavior/Sub-Phase #1/Hough Control/MATLAB Function3 ==
  data: z input; Ox output
function Ox    = C3( z )
%C3 gives the rotation matrix about the z-axis for an angle 'z'
%   z - the angle about the z-axis which you rotate
%   A - the rotation matrix

Ox = [cos(z) sin(z); -sin(z) cos(z)]*[1;0];
end

== matlab function APF_CTL_VIS_Obs_2023a/Phase #3: Experiment/Change BLUE Behavior/Sub-Phase #1/Hough Control/MATLAB Function4 ==
  data: Oy input; e_out output; e_in input
function e_out = fcn(Oy, e_in)

a = sign(Oy'*e_in);
e_out = -a*norm(e_in);

== matlab function APF_CTL_VIS_Obs_2023a/Phase #3: Experiment/Change BLUE Behavior/Sub-Phase #4/Hough Control/MATLAB Function2 ==
  data: Oy output; z input; Ox output
function [Oy, Ox]   = C3( z )
%C3 gives the rotation matrix about the z-axis for an angle 'z'
%   z - the angle about the z-axis which you rotate
%   A - the rotation matrix

Ox = [cos(z) sin(z); -sin(z) cos(z)]*[1;0];
Oy = [cos(z) sin(z); -sin(z) cos(z)]*[0;1];
end

== matlab function APF_CTL_VIS_Obs_2023a/Phase #3: Experiment/Change BLUE Behavior/Sub-Phase #4/Hough Control/MATLAB Function3 ==
  data: z input; Ox output
function Ox    = C3( z )
%C3 gives the rotation matrix about the z-axis for an angle 'z'
%   z - the angle about the z-axis which you rotate
%   A - the rotation matrix

Ox = [cos(z) sin(z); -sin(z) cos(z)]*[1;0];
end

== matlab function APF_CTL_VIS_Obs_2023a/Phase #3: Experiment/Change BLUE Behavior/Sub-Phase #4/Hough Control/MATLAB Function4 ==
  data: Oy input; e_out output; e_in input
function e_out = fcn(Oy, e_in)

a = sign(Oy'*e_in);
e_out = -a*norm(e_in);

== matlab function APF_CTL_VIS_Obs_2023a/Phase #3: Experiment/Change RED Behavior/Sub-Phase #3 /RED_Rz Desired/Wrap/MATLAB Function ==
  data: u input; wrappedAngle output
function wrappedAngle = wrapAngle(u)

wrappedAngle = atan2(sin(u),cos(u));

end

== matlab function APF_CTL_VIS_Obs_2023a/Phase #3: Experiment/Change RED Behavior/Sub-Phase #1/Hough Control/MATLAB Function2 ==
  data: Oy output; z input; Ox output
function [Oy, Ox]   = C3( z )
%C3 gives the rotation matrix about the z-axis for an angle 'z'
%   z - the angle about the z-axis which you rotate
%   A - the rotation matrix

Ox = [cos(z) sin(z); -sin(z) cos(z)]*[1;0];
Oy = [cos(z) sin(z); -sin(z) cos(z)]*[0;1];
end

== matlab function APF_CTL_VIS_Obs_2023a/Phase #3: Experiment/Change RED Behavior/Sub-Phase #1/Hough Control/MATLAB Function3 ==
  data: z input; Ox output
function Ox    = C3( z )
%C3 gives the rotation matrix about the z-axis for an angle 'z'
%   z - the angle about the z-axis which you rotate
%   A - the rotation matrix

Ox = [cos(z) sin(z); -sin(z) cos(z)]*[1;0];
end

== matlab function APF_CTL_VIS_Obs_2023a/Phase #3: Experiment/Change BLUE Behavior/Sub-Phase #2 /Hough Control/MATLAB Function2 ==
  data: Oy output; z input; Ox output
function [Oy, Ox]   = C3( z )
%C3 gives the rotation matrix about the z-axis for an angle 'z'
%   z - the angle about the z-axis which you rotate
%   A - the rotation matrix

Ox = [cos(z) sin(z); -sin(z) cos(z)]*[1;0];
Oy = [cos(z) sin(z); -sin(z) cos(z)]*[0;1];
end

== matlab function APF_CTL_VIS_Obs_2023a/Phase #3: Experiment/Change BLUE Behavior/Sub-Phase #2 /Hough Control/MATLAB Function3 ==
  data: z input; Ox output
function Ox    = C3( z )
%C3 gives the rotation matrix about the z-axis for an angle 'z'
%   z - the angle about the z-axis which you rotate
%   A - the rotation matrix

Ox = [cos(z) sin(z); -sin(z) cos(z)]*[1;0];
end

== matlab function APF_CTL_VIS_Obs_2023a/Phase #3: Experiment/Change BLUE Behavior/Sub-Phase #2 /Hough Control/MATLAB Function4 ==
  data: Oy input; e_out output; e_in input
function e_out = fcn(Oy, e_in)

a = sign(Oy'*e_in);
e_out = -a*norm(e_in);

== matlab function APF_CTL_VIS_Obs_2023a/Phase #3: Experiment/Change RED Behavior/Sub-Phase #1/Hough Control/MATLAB Function4 ==
  data: Oy input; e_out output; e_in input
function e_out = fcn(Oy, e_in)

a = sign(Oy'*e_in);
e_out = -a*norm(e_in);
